simulink model "learn_simuling_control_target_model"  (R2019a)
settings: Solver=VariableStepAuto  StartTime=0.0  StopTime=10.0  RelTol=1e-3
settings Model: Creator=PC  LastModifiedBy=PC

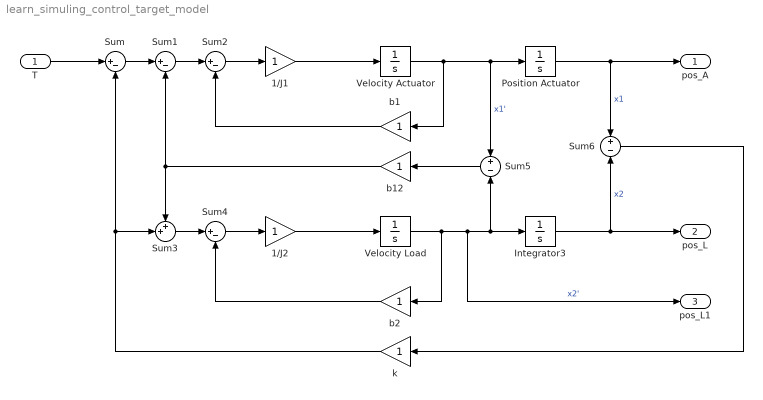
== system learn_simuling_control_target_model ==
  T : Inport
  1/J1 : Gain
  1/J2 : Gain
  Integrator3 : Integrator
  Position Actuator : Integrator
  Sum{,1..2,4} (4 alike) : Sum  Inputs=|+-
  Sum3 : Sum  Inputs=++|
  Sum5 : Sum  Inputs=+|-
  Sum6 : Sum  Inputs=+|-
  Velocity Actuator : Integrator
  Velocity Load : Integrator
  b1 : Gain
  b12 : Gain
  b2 : Gain
  k : Gain
  pos_A : Outport
  pos_L : Outport  Port=2
  pos_L1 : Outport  Port=3
  wires:
  T/1 -> Sum/1
  Sum/1 -> Sum1/1
  Sum1/1 -> Sum2/1
  Sum2/1 -> 1/J1/1
  1/J1/1 -> Velocity Actuator/1
  Velocity Actuator/1 -> b1/1, Position Actuator/1, Sum5/1  "x1'"
  Position Actuator/1 -> Sum6/1, pos_A/1  "x1"
  b1/1 -> Sum2/2
  Sum5/1 -> b12/1
  b12/1 -> Sum3/1, Sum1/2
  Sum3/1 -> Sum4/1
  Sum4/1 -> 1/J2/1
  1/J2/1 -> Velocity Load/1
  Velocity Load/1 -> b2/1, pos_L1/1, Sum5/2, Integrator3/1  "x2'"
  b2/1 -> Sum4/2
  Integrator3/1 -> Sum6/2, pos_L/1  "x2"
  Sum6/1 -> k/1
  k/1 -> Sum3/2, Sum/2
